simulink model "simula"  (R2025b)
settings: Solver=ode4  StartTime=0.0  StopTime=10  FixedStep=0.001  RelTol=1e-3
InitFcn:
  | run("init.m")
undefined symbols (not defined in the file or in its folder): robot_params
settings Model: Creator=aldor  LastModifiedBy=aldor

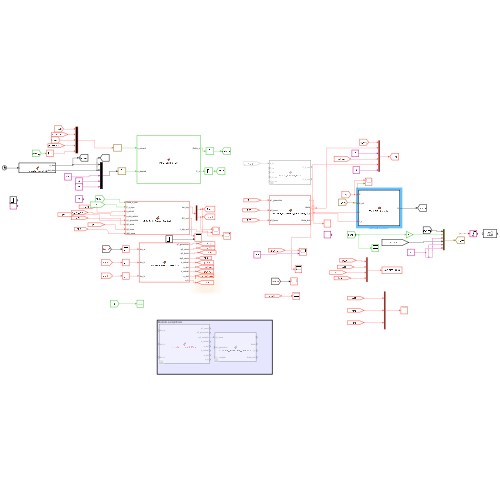
[thumbnail: Simulink's stored preview of the top-level diagram]
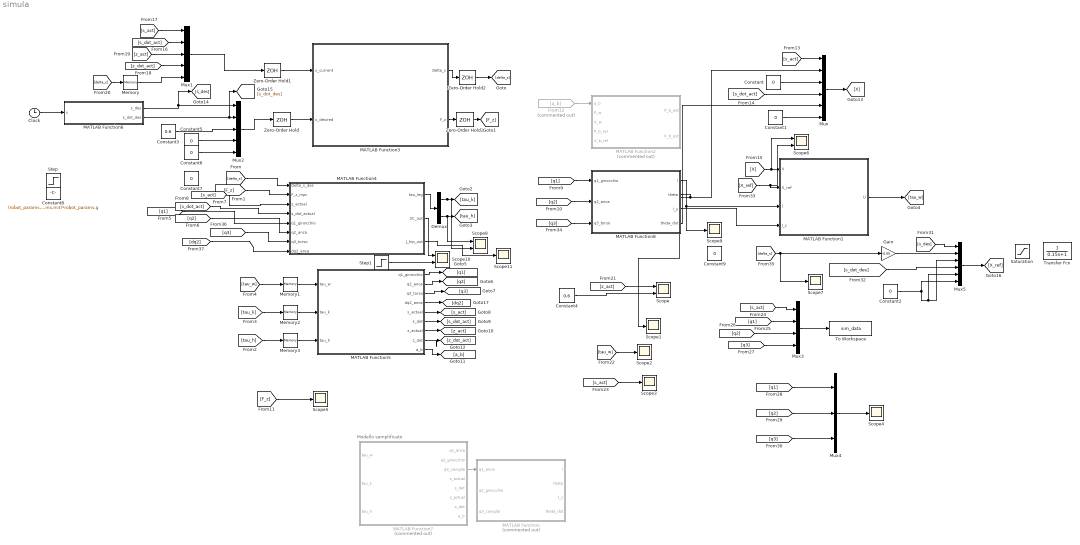
== system simula ==
  note: Modello semplificato
  Clock : Clock
  Constant{,1..2,5..7,9} (7 alike) : Constant  Value=0
  Constant3 : Constant  Value=0.6
  Constant4 : Constant  Value=0.6
  Constant8 : Constant  Value=(robot_params.m1+robot_params.m2+robot_params.m3)*robot_params.g
  Demux : Demux  Outputs=2
  From12 : From  Commented=on  GotoTag=a_b
  Gain : Gain  Gain=-0.05
  MATLAB Function : MATLAB Function  Commented=on  TreatAsAtomicUnit=on
  MATLAB Function1 : MATLAB Function  TreatAsAtomicUnit=on
  MATLAB Function2 : MATLAB Function  Commented=on  TreatAsAtomicUnit=on
  MATLAB Function3 : MATLAB Function  TreatAsAtomicUnit=on
  MATLAB Function4 : MATLAB Function  TreatAsAtomicUnit=on
  MATLAB Function5 : MATLAB Function  TreatAsAtomicUnit=on
  MATLAB Function6 : MATLAB Function  TreatAsAtomicUnit=on
  MATLAB Function7 : MATLAB Function  Commented=on  TreatAsAtomicUnit=on
  MATLAB Function8 : MATLAB Function  TreatAsAtomicUnit=on
  Memory{,1..3} (4 alike) : Memory
  Mux : Mux  Inputs=6
  Mux1 : Mux  Inputs=5
  Mux2 : Mux  Inputs=5
  Mux3 : Mux
  Mux4 : Mux  Inputs=3
  Mux5 : Mux  Inputs=6
  Saturation : Saturate  UpperLimit=0.15  LowerLimit=-0.15
  Scope{,6,8,10} (4 alike) : Scope  NumInputPorts=2
      Scope settings: ActiveDisplayYMinimum=0.1067548531401226  ActiveDisplayYMaximum=0.98813834965109748
      Scope10 settings: ActiveDisplayYMinimum=-0.10648253135574463  ActiveDisplayYMaximum=0.077550360917162844  DataLoggingVariableName=ScopeData10
      Scope6 settings: ActiveDisplayYMinimum=-1  ActiveDisplayYMaximum=1  DataLoggingVariableName=ScopeData6
      Scope8 settings: ActiveDisplayYMinimum=-188.72850710541874  ActiveDisplayYMaximum=1090.9634519642959  DataLoggingVariableName=ScopeData8
  Scope{1..5,7,9,11} (8 alike) : Scope
      Scope1 settings: ActiveDisplayYMinimum=-0.026598662061855207  ActiveDisplayYMaximum=0.032394796278817736
      Scope11 settings: ActiveDisplayYMinimum=-0.97377388155977385  ActiveDisplayYMaximum=0.0650927535868372  DataLoggingVariableName=ScopeData11
      Scope2 settings: ActiveDisplayYMinimum=-11.512015900207867  ActiveDisplayYMaximum=2.9564436285874827  DataLoggingVariableName=ScopeData2
      Scope3 settings: ActiveDisplayYMinimum=-0.15390799680390416  ActiveDisplayYMaximum=1.2448530557444439  DataLoggingVariableName=ScopeData3
      Scope4 settings: ActiveDisplayYMinimum=-3.0379257120480285  ActiveDisplayYMaximum=0.34452501241406891  DataLoggingVariableName=ScopeData4
      Scope5 settings: ActiveDisplayYMinimum=-792.61159771990333  ActiveDisplayYMaximum=837.79442871292474  DataLoggingVariableName=ScopeData5
      Scope7 settings: ActiveDisplayYMinimum=-49.518935737152816  ActiveDisplayYMaximum=5.69391944382371  DataLoggingVariableName=ScopeData7
      Scope9 settings: ActiveDisplayYMinimum=0.26491553159842146  ActiveDisplayYMaximum=1.1125448908081954  DataLoggingVariableName=ScopeData9
  Step : Step  Time=2  After=0.05  SampleTime=0
  Step1 : Step  Time=2  After=0.05  SampleTime=0
  To Workspace : ToWorkspace  VariableName=sim_data  SampleTime=-1
  Transfer Fcn : TransferFcn  Denominator=[0.15 1]
  Zero-Order Hold{,1..3} (4 alike) : ZeroOrderHold  SampleTime=1e-2
  wires:
  MATLAB Function4/1(tau_leg) -> Demux/1
  Demux/1 -> Scope8/2, [tau_k]
  Demux/2 -> Scope8/1, [tau_h]
  MATLAB Function1/1(U) -> [tau_w]
  MATLAB Function8/1(l) -> Scope9/1, MATLAB Function1/3(l)
  MATLAB Function8/3(I_y) -> MATLAB Function1/4(I_y)
  MATLAB Function5/1(q1_ginocchio) -> [q1]
  MATLAB Function5/2(q2_anca) -> [q2]
  MATLAB Function5/3(q3_torso) -> [q3]
  MATLAB Function5/7(z_actual) -> [z_act]
  MATLAB Function5/5(s_actual) -> [s_act]
  MATLAB Function5/6(s_dot) -> [s_dot_act]
  MATLAB Function5/8(z_dot) -> [z_dot_act]
  MATLAB Function5/9(a_b) -> [a_b]
  [s_act] -> MATLAB Function4/3(s_actual)
  [s_dot_act] -> MATLAB Function4/4(s_dot_actual)
  [q2] -> MATLAB Function8/2(q2_anca)
  [q1] -> MATLAB Function8/1(q1_ginocchio)
  [q3] -> MATLAB Function8/3(q3_torso)
  From12/1 -> MATLAB Function2/1(a_b)
  [s_act] -> Mux/1
  Constant/1 -> Mux/3
  MATLAB Function8/2(theta) -> Scope1/1, Mux/2
  [s_dot_act] -> Mux/4
  Constant1/1 -> Mux/6
  Mux/1 -> [X]
  [X] -> Scope6/1, MATLAB Function1/1(X)
  [X_ref] -> Scope6/2, MATLAB Function1/2(X_ref)
  [s_dot_act] -> Mux1/2
  [s_act] -> Mux1/1
  [z_act] -> Mux1/3
  [z_dot_act] -> Mux1/4
  [delta_s] -> Memory/1
  Memory/1 -> Mux1/5
  Constant5/1 -> Mux2/4
  Constant6/1 -> Mux2/5
  [tau_w] -> Memory1/1
  Memory1/1 -> MATLAB Function5/1(tau_w)
  Memory2/1 -> MATLAB Function5/2(tau_k)
  [tau_k] -> Memory2/1
  [tau_h] -> Memory3/1
  Memory3/1 -> MATLAB Function5/3(tau_h)
  [z_act] -> Scope/1
  Constant4/1 -> Scope/2
  [tau_w] -> Scope2/1
  [s_act] -> Scope3/1
  Mux3/1 -> To Workspace/1
  [s_act] -> Mux3/1
  [q1] -> Mux3/2
  [q2] -> Mux3/3
  [q3] -> Mux3/4
  [q2] -> Mux4/2
  [q3] -> Mux4/3
  [q1] -> Mux4/1
  Mux4/1 -> Scope4/1
  MATLAB Function8/4(theta_dot) -> Mux/5
  Clock/1 -> MATLAB Function6/1(t)
  MATLAB Function6/1(s_des) -> [s_des], Mux2/1
  MATLAB Function6/2(s_dot_des) -> [s_dot_des], Mux2/2
  Constant3/1 -> Mux2/3
  [s_des] -> Mux5/1
  Constant2/1 -> Mux5/5, Mux5/3, Mux5/6
  [s_dot_des] -> Mux5/4
  Mux5/1 -> [X_ref]
  [F_z] -> Scope5/1
  [F_z] -> MATLAB Function4/2(F_z_mpc)
  ? -> Saturation/1
  [delta_s] -> Gain/1, Scope7/1
  Gain/1 -> Mux5/2
  Mux2/1 -> Zero-Order Hold/1
  Zero-Order Hold/1 -> MATLAB Function3/2(x_desired)
  Zero-Order Hold1/1 -> MATLAB Function3/1(x_current)
  Mux1/1 -> Zero-Order Hold1/1
  Zero-Order Hold2/1 -> [delta_s]
  MATLAB Function3/1(Delta_s) -> Zero-Order Hold2/1
  MATLAB Function3/2(F_z) -> Zero-Order Hold3/1
  Zero-Order Hold3/1 -> [F_z]
  MATLAB Function7/3(q3_caviglia) -> MATLAB Function/1(q1_anca)
  [delta_s] -> MATLAB Function4/1(Delta_s_des)
  MATLAB Function5/4(dq2_anca) -> [dq2]
  [q3] -> MATLAB Function4/7(q3_torso)
  [dq2] -> MATLAB Function4/8(dq2_anca)
  MATLAB Function4/2(SC_out) -> Scope10/1
  Step1/1 -> Scope10/2
  MATLAB Function4/3(J_hip_out) -> Scope11/1
  [q2] -> MATLAB Function4/6(q2_anca)
  [q1] -> MATLAB Function4/5(q1_ginocchio)

== matlab function simula/MATLAB Function7 ==
  data: tau_w input; q1_anca output; tau_k input; tau_h input; q2_ginocchio output; q3_caviglia output; s_actual output; s_dot output; z_actual output; z_dot output; a_b output
function [q1_anca, q2_ginocchio, q3_caviglia, s_actual, s_dot, z_actual, z_dot, a_b] = Simulated_Robot_Plant(tau_w, tau_k, tau_h)
    q1_anca = 0.0; q2_ginocchio = 0.0; q3_caviglia = 0.0;
    s_actual = 0.0; s_dot = 0.0; z_actual = 0.0; z_dot = 0.0;
    a_b = zeros(2,1);

    persistent X_z X_wip
    if isempty(X_z)
        X_z = [0.6; 0];       
        X_wip = [0; 0; 0; 0]; 
    end
    dt = 0.001; g = 9.81; m_b = 73.0; r = 0.127; m_w = 3.5; I_w = 0.1; l = 0.45;

    %% 1. FISICA VERTICALE (Z)
    ratio = X_z(1) / (2*l);
    if ratio > 0.999, ratio = 0.999; elseif ratio < -0.999, ratio = -0.999; end
    q2_current = 2 * acos(ratio);
    
    J_z_knee = -l * sin(q2_current / 2);
    if abs(J_z_knee) < 0.05, J_z_knee = -0.05 * sign(q2_current + 1e-6); end
    
    F_z_applied = tau_k / J_z_knee; 
    z_ddot = (F_z_applied / m_b) - g;
    
    X_z(2) = X_z(2) + z_ddot * dt;
    X_z(1) = X_z(1) + X_z(2) * dt;
    
    % Blocchi fisici estremi per evitare decolli o sprofondamenti
    if X_z(1) < 0.2, X_z(1) = 0.2; X_z(2) = 0; end 
    if X_z(1) > 0.9, X_z(1) = 0.9; X_z(2) = 0; end 
    z_act = X_z(1);

    %% 2. FISICA DEL PENDOLO Orizzontale
    l_pend = z_act;
    if l_pend > 0.9, l_pend = 0.9; end 
    if l_pend < 0.1, l_pend = 0.1; end
    
    I_y = (1/3) * m_b * l_pend^2;

    D = 2*I_w*(I_y + m_b*l_pend^2) + (2*l_pend^2*m_b*m_w + I_y*(m_b + 2*m_w)*r^2);
    a1 = -(g * l_pend^2 * m_b^2 * r^2) / D;
    a2 =  (g * l_pend * m_b * (2*I_w + (m_b + 2*m_w)*r^2)) / D;
    b1 =  (r * (I_y + l_pend*m_b*(l_pend + r))) / D;
    b2 = -(2*I_w + r*(l_pend*m_b + (m_b + 2*m_w)*r)) / D;

    A_wip = [0 0 1 0; 0 0 0 1; 0 a1 0 0; 0 a2 0 0];
    B_wip = [0 0; 0 0; b1 b1; b2 b2];

    % LA CORREZIONE VITALE: Diamo ai motori la forza di bilanciare 73 kg!
    tau_w_lim = tau_w;
    limite = 1000; % Aumentato da 15 a 1000 Nm
    if tau_w_lim(1) > limite, tau_w_lim(1) = limite; end
    if tau_w_lim(1) < -limite, tau_w_lim(1) = -limite; end
    if tau_w_lim(2) > limite, tau_w_lim(2) = limite; end
    if tau_w_lim(2) < -limite, tau_w_lim(2) = -limite; end

    X_wip_dot = A_wip * X_wip + B_wip * tau_w_lim;
    X_wip = X_wip + X_wip_dot * dt;
    theta_vero = X_wip(2);

    %% 3. ASSEGNAZIONE GIUNTI (La tua convenzione perfetta)
    ratio_new = z_act / (2*l);
    if ratio_new > 0.999, ratio_new = 0.999; elseif ratio_new < -0.999, ratio_new = -0.999; end
    q2_ginocchio = 2 * acos(ratio_new);
    
    alpha = q2_ginocchio / 2;
    q3_caviglia = -alpha + theta_vero;
    q1_anca = -alpha;

    %% 4. ASSEGNAZIONE USCITE
    s_actual = X_wip(1);
    s_dot = X_wip(3);
    z_actual = z_act;
    z_dot = X_z(2);
    a_b = [X_wip_dot(3); z_ddot + g];
end

== matlab function simula/MATLAB Function8 ==
  data: q1_ginocchio input; l output; q2_anca input; q3_torso input; theta output; I_y output; theta_dot output
function [l, theta, I_y, theta_dot] = calculate_equivalent_pendulum_v3(q1_ginocchio, q2_anca, q3_torso)
    persistent theta_prev
    if isempty(theta_prev), theta_prev = 0; end
    dt = 0.001;

    m1=1.2; m2=5.3; m3=60.0;
    l1=0.45; l2=0.45; l3=0.35;

    phi_shank = q1_ginocchio - q2_anca + q3_torso;
    phi_thigh = q3_torso - q2_anca;

    x1 = (l1/2)*sin(phi_shank);              y1 = (l1/2)*cos(phi_shank);
    xk = l1*sin(phi_shank);                  yk = l1*cos(phi_shank);
    x2 = xk + (l2/2)*sin(phi_thigh);         y2 = yk + (l2/2)*cos(phi_thigh);
    xh = xk + l2*sin(phi_thigh);             yh = yk + l2*cos(phi_thigh);
    x3 = xh + (l3/2)*sin(q3_torso);          y3 = yh + (l3/2)*cos(q3_torso);

    m_tot = m1+m2+m3;
    SC = (m1*x1 + m2*x2 + m3*x3) / m_tot;
    ZC = (m1*y1 + m2*y2 + m3*y3) / m_tot;

    l = sqrt(SC^2 + ZC^2);
    if l < 0.1, l = 0.1; end

    theta = atan2(SC, ZC);

    % Unwrap per evitare i falsi picchi di theta_dot
    delta_theta = theta - theta_prev;
    delta_theta = atan2(sin(delta_theta), cos(delta_theta));
    theta_dot = delta_theta / dt;
    theta_prev = theta;

    I_y = (1/3) * m_tot * l^2;
end

== matlab function simula/MATLAB Function1 ==
  data: X input; U output; X_ref input; l input; I_y input
function U = TV_LQR_Controller(X, X_ref, l, I_y)
    % X: Stato attuale [s; theta; phi; s_dot; theta_dot; phi_dot] (6x1)
    % X_ref: Stato target desiderato [s_ref; theta_ref; phi_ref; 0; 0; 0] (6x1)
    % l: Lunghezza attuale del pendolo equivalente [m]
    % I_y: Inerzia attuale del corpo superiore [kg*m^2]
    
    % Per usare la funzione lqr() di MATLAB all'interno di Simulink, 
    % dobbiamo dichiararla come estrinseca.
    coder.extrinsic('lqr');
    if l < 0.1
        l = 0.1;
    end
    if I_y < 1e-3
        I_y = 1e-3;
    end
    % 1. Richiamo Parametri Fisici
    m_w = 3.5;       % Massa ruota
    I_w = 0.1;       % Inerzia ruota
    r   = 0.127;     % Raggio ruota
    d   = 0.63;      % Distanza ruote
    m_b = 73.0;      % Massa corpo superiore
    I_z = 3.3;       % Inerzia torso asse z
    g   = 9.81;      % Gravità
    
    % 2. Calcolo dei Coefficienti della Dinamica (Eq. 14)
    % Denominatore comune per a1, a2, b1, b2
    D = 2*I_w*(I_y + m_b*l^2) + (2*l^2*m_b*m_w + I_y*(m_b + 2*m_w)*r^2);
    
    a1 = -(g * l^2 * m_b^2 * r^2) / D;
    a2 =  (g * l * m_b * (2*I_w + (m_b + 2*m_w)*r^2)) / D;
    
    b1 =  (r * (I_y + l*m_b*(l + r))) / D;
    b2 = -(2*I_w + r*(l*m_b + (m_b + 2*m_w)*r)) / D;
    
    % Coefficiente disaccoppiato per lo steering (imbardata)
    b3 =  (d * r) / (2*I_z*r^2 + d^2*(I_w + m_w*r^2));
    
    % 3. Costruzione Matrici di Stato A(l) e Input B(l) (Eq. 12, Eq. 13)
    A = zeros(6, 6);
    A(1, 4) = 1; 
    A(2, 5) = 1; 
    A(3, 6) = 1;
    A(4, 2) = a1;
    A(5, 2) = a2;
    
    B = zeros(6, 2);
    B(4, 1) = b1;  B(4, 2) = b1;
    B(5, 1) = b2;  B(5, 2) = b2;
    B(6, 1) = b3;  B(6, 2) = -b3;
    
    % 4. Definizione Matrici di Peso Q e R (Tuning LQR)
    % Questi valori determinano l'aggressività del controllore. 
    % Possono essere trasformati in input del blocco per un tuning rapido.
    % 4. Definizione Matrici di Peso Q e R (Tuning Soft)
    % Pesi drasticamente ridotti per evitare instabilità con il ritardo discreto
% Aumenta il peso sugli angoli (q1, q2) per evitare che saturino
%X = [s, θ, φ, ṡ, θ̇, φ̇]
    Q = diag([50, 50, 100, 50, 10, 1]);
    R = diag([1, 1]) * 0.5;         % uso coppie piu abbasso piu accelera
    
    % 5. Risoluzione LQR e Calcolo Input
    % Inizializza K per la Code Generation di Simulink
    K = zeros(2, 6); 
    
    % Calcola la matrice dei guadagni ottimali K
    K = lqr(A, B, Q, R);
    
    % Errore di stato (tilde_X)
    X_tilde = X - X_ref;
    
    % Legge di controllo finale (Eq. 16): U = [tau_l; tau_r]
    U = -K * X_tilde; 
end

== matlab function simula/MATLAB Function ==
  data: q1_anca input; l output; q2_ginocchio input; q3_caviglia input; theta output; I_y output; theta_dot output
function [l, theta, I_y, theta_dot] = calculate_equivalent_pendulum(q1_anca, q2_ginocchio, q3_caviglia)
    persistent theta_prev
    if isempty(theta_prev), theta_prev = 0; end
    dt = 0.001;

    % Somma degli angoli della catena
    theta = q1_anca + q2_ginocchio + q3_caviglia;
    theta_dot = (theta - theta_prev) / dt;
    theta_prev = theta;

    l = 2 * 0.45 * cos(q2_ginocchio / 2);
    if l < 0.1, l = 0.1; end
    m_b = 73.0;
    I_y = (1/3) * m_b * l^2;
end

== matlab function simula/MATLAB Function2 ==
  data: a_b input; P_b_est output; P_w input; V_w input; P_b_rel input; V_b_rel input; V_b_est output
function [P_b_est, V_b_est] = Linear_Kalman_Filter(a_b, P_w, V_w, P_b_rel, V_b_rel)
    % INGRESSI:
    % a_b: Accelerazione del torso misurata dall'IMU [2x1] (asse s, asse z)
    % P_w: Posizione dell'asse ruote (odometria) [2x1]
    % V_w: Velocità dell'asse ruote (odometria) [2x1]
    % P_b_rel: Posizione del torso rispetto all'asse (cinematica diretta) [2x1]
    % V_b_rel: Velocità del torso rispetto all'asse (jacobiano gambe) [2x1]
    
    % Definisci dt (Tempo di campionamento, es. 1000 Hz dal paper)
    dt = 0.001; 
    
    % Variabili di stato persistenti per mantenere la memoria tra i loop di Simulink
    persistent X P
    if isempty(X)
        X = zeros(4, 1); % Stato [Posizione_s; Posizione_z; Velocità_s; Velocità_z]
        P = eye(4);      % Matrice di covarianza dell'errore iniziale
    end
    
    % 1. Matrici del Modello (Eq. 20 e 21)
    I2 = eye(2);
    O2 = zeros(2, 2);
    
    A = [I2, dt*I2; 
         O2, I2];
         
    B = [O2; 
         dt*I2];
         
    H = [I2, O2; 
         O2, I2];
         
    % 2. Matrici di Covarianza del Rumore (Da calibrare sul sistema reale)
    Q = eye(4) * 0.01;  % Rumore di processo (incertezza del modello)
    R = eye(4) * 0.1;   % Rumore di misura (incertezza dei sensori)
    
    % Nota dal paper: durante il salto, il rumore di osservazione (R) 
    % andrebbe aumentato perché l'encoder della ruota perde di affidabilità.
    
    % --- FASE 1: PREDIZIONE (PREDICT) ---
    % Previsione dello stato basata sull'accelerazione dell'IMU (Eq. 20)
    X_pred = A * X + B * a_b;
    P_pred = A * P * A' + Q;
    
    % --- FASE 2: AGGIORNAMENTO (UPDATE) ---
    % Costruzione della misurazione Z (Eq. 21)
    % Z contiene la posizione assoluta (Ruota + Relativa) e velocità
    Z = [P_w + P_b_rel; 
         V_w + V_b_rel];
    
    % Calcolo del guadagno di Kalman
    S = H * P_pred * H' + R;
    K_kalman = P_pred * H' / S;
    
    % Aggiornamento dello stato stimato e della covarianza
    X = X_pred + K_kalman * (Z - H * X_pred);
    P = (eye(4) - K_kalman * H) * P_pred;
    
    % USCITE: Estrazione di Posizione e Velocità stimate
    P_b_est = X(1:2);
    V_b_est = X(3:4);
end

== matlab function simula/MATLAB Function3 ==
  data: x_current input; Delta_s output; x_desired input; F_z output
function [Delta_s, F_z] = MPC_Custom_QP(x_current, x_desired)
    % quadprog non è supportato nativamente per la code generation C
    coder.extrinsic('quadprog');
    coder.extrinsic('optimoptions');

    %% 1. Parametri e Discretizzazione
    m_b = 73.0; 
    g = 9.81;    
    
    h = x_current(3); 
    if h < 0.1
        h = 0.6;
    end
    
    dt = 0.01; 
    N = 40;     
    
    A_c = zeros(5,5);
    A_c(1,2) = 1;
    A_c(3,4) = 1;
    A_c(2,5) = g / h; 
    
    B_c = zeros(5,2);
    B_c(4,2) = 1 / m_b;
    B_c(5,1) = 1;
    
    A_d = eye(5) + A_c * dt;
    B_d = B_c * dt;

    %% 2. Pesi della Funzione di Costo
    %x = [s, ṡ, z, ż, Δs]
    S = diag([1, 1, 500, 50, 1]);
    W = diag([1, 0.01]);

    %% 3. Condensazione (Srotolamento) 
    nx = 5; nu = 2;
    P_x = zeros(nx*N, nx);
    P_u = zeros(nx*N, nu*N);

    A_power = eye(nx);
    for i = 1:N
        A_power = A_power * A_d;
        P_x((i-1)*nx+1 : i*nx, :) = A_power;
        for j = 1:i
            P_u((i-1)*nx+1 : i*nx, (j-1)*nu+1 : j*nu) = (A_d^(i-j)) * B_d;
        end
    end

    S_bar = kron(eye(N), S);
    W_bar = kron(eye(N), W);

    H = 2 * (P_u' * S_bar * P_u + W_bar);
    H = (H + H') / 2; % Garantisce simmetria perfetta
    
    X_ref = repmat(x_desired, N, 1);
    f = 2 * P_u' * S_bar * (P_x * x_current - X_ref);

    %% 4. Vincoli Fisici
    F_min = -1500; % Permette di frenare!
    F_max = 1500;
    
    LB = zeros(nu*N, 1);
    UB = zeros(nu*N, 1);
    
    for i = 1:N
        LB((i-1)*nu+1) = -0.20;   % era -2.0

        UB((i-1)*nu+1) =  0.20;   % era  2.0
 
        
        LB((i-1)*nu+2) = F_min; 
        UB((i-1)*nu+2) = F_max;
    end

    %% 5. Risoluzione QP (CORRETTA)
    % Pre-allocazione per Simulink Coder
    U_opt_calc = zeros(nu*N, 1);
    fval = 0.0;
    exitflag = 0.0;
    
    % Algoritmo robusto di default
    options = optimoptions('quadprog', 'Display', 'off');
    
    % LA CORREZIONE: Aggiunto "fval" per non sballare "exitflag"!
    [U_opt_calc, fval, exitflag] = quadprog(H, f, [], [], [], [], LB, UB, [], options);

    if exitflag > 0
        U_opt = U_opt_calc;
    else
        % Se fallisce davvero, eroga 0 extra, ma il VMC ci terrà in piedi col peso base
        U_opt = zeros(nu*N, 1);
    end

    %% 6. Estrazione Input Ottimo
    Delta_s_dot_opt = U_opt(1);
    F_z = U_opt(2); % FINALMENTE SARA' DIVERSO DA ZERO!

    Delta_s = x_current(5) + Delta_s_dot_opt * dt;
end

== matlab function simula/MATLAB Function4 ==
  settings: updateMethod=DISCRETE
  data: Delta_s_des input; tau_leg output; F_z_mpc input; s_actual input; s_dot_actual input; SC_out output; J_hip_out output; q1_ginocchio input; q2_anca input; q3_torso input; dq2_anca input
function [tau_leg, SC_out, J_hip_out] = VMC_Task_Space_Controller(Delta_s_des, F_z_mpc, s_actual, s_dot_actual, ...
                                               q1_ginocchio, q2_anca, q3_torso, dq2_anca)

% =========================================================================

% VMC CORRETTO - Ripartizione pulita delle competenze della GAMBA:

%   GINOCCHIO -> altezza z          (canale verticale)

%   ANCA      -> beccheggio torso q3 (stabilizzazione, anello prima mancante)

% Lo spostamento ORIZZONTALE del CoM NON e' piu' gestito qui: e' compito

% della ruota (TV-LQR). Cosi' sparisce il conflitto che destabilizzava l'MPC.

%

% Delta_s_des, s_actual, s_dot_actual, dq2_anca restano solo per compatibilita'

% di cablaggio (non sono piu' usati per il controllo dell'anca).

% =========================================================================
 
    % --- Uscite inizializzate (necessario per code generation) ---

    tau_leg   = zeros(2,1);

    SC_out    = 0.0;

    J_hip_out = 0.0;
 
    % --- Parametri fisici ---

    l1 = 0.45; l2 = 0.45;

    z_des = 0.6;          % altezza di equilibrio (asse ruota -> anca) [m]

    dt    = 0.001;        % deve coincidere col passo fisso del solutore
 
    % --- Stima derivate via differenza finita (persistenti) ---

    persistent q3_prev z_prev

    if isempty(q3_prev), q3_prev = q3_torso; end
 
    % Cinematica utile

    phi_shank = q1_ginocchio - q2_anca + q3_torso;

    phi_thigh = q3_torso - q2_anca;

    z_actual  = l1*cos(phi_shank) + l2*cos(phi_thigh);
 
    if isempty(z_prev), z_prev = z_actual; end
 
    dq3   = (q3_torso - q3_prev)/dt;   q3_prev = q3_torso;

    z_dot = (z_actual - z_prev)/dt;    z_prev  = z_actual;
 
    % --- CoM: solo per monitoraggio/uscite ---

    coder.extrinsic('calc_com_jacobian');

    J_SC = zeros(1,2); J_ZC = zeros(1,2); SC = 0.0; ZC = 0.0;

    [J_SC, J_ZC, SC, ZC] = calc_com_jacobian(q1_ginocchio, q2_anca, q3_torso);

    SC_out    = SC;

    J_hip_out = J_SC(2);
 
    % --- Compensazione di gravita' dalla dinamica VERA G(q) ---

    % (sostituisce il vecchio Jacobiano del ginocchio "clampato", instabile

    %  a gamba dritta). G non dipende da dq, quindi passo dq = 0.

    coder.extrinsic('calc_dynamics');

    q_full  = [q1_ginocchio; 0; q2_anca; q3_torso];   % ordine [q1;qw;q2;q3]

    M   = zeros(4,4); CdQ = zeros(4,1); G = zeros(4,1);

    [M, CdQ, G] = calc_dynamics(q_full, zeros(4,1));

    tau_k_grav = G(1);   % coppia statica ginocchio

    tau_h_grav = G(3);   % coppia statica anca
 
    % =====================================================================

    % (1) GINOCCHIO  ->  controllo di ALTEZZA

    % =====================================================================

    Kp_z = 4000; Kd_z = 300;               % PD altezza (DA TARARE)

    Jz_knee = -l1*sin(phi_shank);          % dz/dq1

    if abs(Jz_knee) < 0.05                  % vicino a gamba dritta: autorita' ~0

        Jz_knee = 0.05*sign(Jz_knee + 1e-9);

    end

    F_z_cmd = Kp_z*(z_des - z_actual) - Kd_z*z_dot + F_z_mpc;  % forza vert. extra

    tau_k   = tau_k_grav + Jz_knee * F_z_cmd;
 
    % =====================================================================

    % (2) ANCA  ->  stabilizza il BECCHEGGIO del torso  q3 -> 0

    % =====================================================================

    Kp_t = 800; Kd_t = 80;                 % PD torso (DA TARARE)

    % SEGNO: parti con -(Kp*q3 + Kd*dq3). Se in simulazione il torso DIVERGE

    %        invece di raddrizzarsi, INVERTI il segno del termine PD.

    tau_h = tau_h_grav - (Kp_t*q3_torso + Kd_t*dq3);
 
    tau_leg = [tau_k; tau_h];

end

== matlab function simula/MATLAB Function5 ==
  data: tau_w input; q1_ginocchio output; tau_k input; tau_h input; q2_anca output; q3_torso output; dq2_anca output; s_actual output; s_dot output; z_actual output; z_dot output; a_b output
function [q1_ginocchio, q2_anca, q3_torso, dq2_anca, s_actual, s_dot, z_actual, z_dot, a_b] = ...
          Simulated_Robot_Plant_Full(tau_w, tau_k, tau_h)

    q1_ginocchio = 0.0; q2_anca = 0.0; q3_torso = 0.0; dq2_anca = 0.0;
    s_actual = 0.0; s_dot = 0.0; z_actual = 0.0; z_dot = 0.0;
    a_b = zeros(2,1);

    persistent q dq
    if isempty(q)
        q  = [0; 0; 0; 0];
        dq = [0; 0; 0; 0];
    end

    dt = 0.001;
    limite_ruota = 50; limite_gamba = 300;
    tau_w_scalar = max(min(tau_w(1)+tau_w(2), limite_ruota), -limite_ruota);
    tau_k_lim    = max(min(tau_k, limite_gamba), -limite_gamba);
    tau_h_lim    = max(min(tau_h, limite_gamba), -limite_gamba);

    tau_vec = [tau_k_lim; tau_w_scalar; tau_h_lim; 0];

    ddq = whole_robot_2D(q, dq, tau_vec);
    dq  = dq + ddq * dt;
    q   = q  + dq * dt;

    q1_ginocchio = q(1);
    q2_anca      = q(3);
    q3_torso     = q(4);
    dq2_anca     = dq(3);        % <-- nuova uscita

    Rw = 0.127;
    s_actual = Rw * q(2);
    s_dot    = Rw * dq(2);

    l1 = 0.45; l2 = 0.45;
    phi_shank = q1_ginocchio - q2_anca + q3_torso;
    phi_thigh = q3_torso - q2_anca;
    z_actual = l1*cos(phi_shank) + l2*cos(phi_thigh);

    persistent z_prev
    if isempty(z_prev), z_prev = z_actual; end
    z_dot = (z_actual - z_prev)/dt;
    z_prev = z_actual;

    a_b = [ddq(2)*Rw; z_dot];
end

== matlab function simula/MATLAB Function6 ==
  data: t input; s_des output; s_dot_des output
function [s_des, s_dot_des] = Smooth_Trajectory(t)
    % PRE-ALLOCAZIONE PER IL CODER
    s_des = 0.0;
    s_dot_des = 0.0;
    
    % PARAMETRI DELLA TRAIETTORIA
    t_start = 0.0;       % Il robot inizia a muoversi a 2 secondi
    t_end = 5.0;         % Arriva a destinazione a 5 secondi (3 secondi di viaggio)
    s_final = 1.0;       % Destinazione orizzontale (1 metro)
    
    % LOGICA DEL MOVIMENTO
    if t <= t_start
        % Prima di partire, resta fermo
        s_des = 0.0;
        s_dot_des = 0.0;
        
    elseif t >= t_end
        % Arrivato a destinazione, fermati
        s_des = s_final;
        s_dot_des = 0.0;
        
    else
        % FASE DI MOTO: Polinomio Cubico (Minimum Jerk Trajectory)
        % Normalizziamo il tempo tra 0 e 1 per la durata del viaggio
        tau = (t - t_start) / (t_end - t_start);
        
        % Posizione (Profilo a "S" morbida)
        s_des = s_final * (3*tau^2 - 2*tau^3);
        
        % Velocità (Derivata della posizione, forma a campana)
        s_dot_des = s_final * (6*tau - 6*tau^2) / (t_end - t_start);
    end
end
